simulink model "ExperimentalPowertrain"  (R2019b)
settings: Solver=ode1  StartTime=0.0  StopTime=inf  FixedStep=0.0002  RelTol=1e-3
PreLoadFcn:
  | vehicle = 'Car'; if ~length(which('cmself')), cmenv; end
  | ExperimentalPowertrain_bus
InitFcn:
  | vehicle = 'Car'; if ~length(which('cmself')), cmenv; end
  | ExperimentalPowertrain_bus
libraries: CarMaker4SL x8
(part 1 of 2)
Description:
  | CarMaker Plug-in Model Target
settings Model: Creator=caleb  LastModifiedBy=caleb
settings RTWCC: Description=CarMaker Plug-in Model Target  SystemTargetFile=CarMaker.tlc  TemplateMakefile=CarMaker_unix-win64.tmf
settings CodeAppCC: MaxIdLength=127
settings STFCustomTargetCC: TargetLangStandard=C99 (ISO)  CombineOutputUpdateFcns=on  MultiInstanceERTCode=on  CodeInterfacePackaging=Reusable function  GenerateAllocFcn=on  SystemTargetFile=CarMaker.tlc
settings GRTTargetCC: ParMdlRefBuildCompliant=off  CompOptLevelCompliant=off  ConcurrentExecutionCompliant=off  MatFileLogging=off  MultiInstanceERTCode=on  CodeInterfacePackaging=Reusable function  CPPClassGenCompliant=off  GenerateAllocFcn=on  UseToolchainInfoCompliant=off

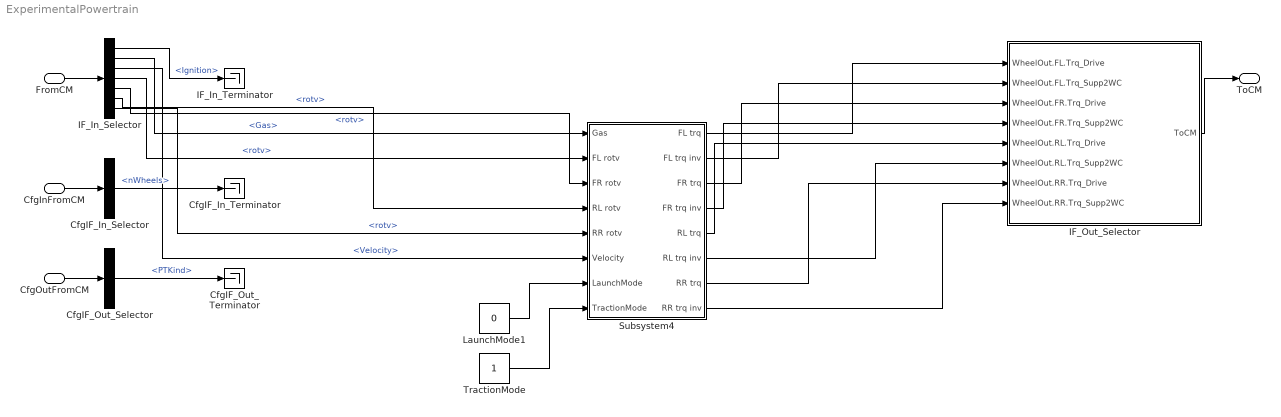
== system ExperimentalPowertrain ==
  FromCM : Inport  OutDataTypeStr=Bus: cmPowerTrainXWDIn
  CfgInFromCM : Inport  Port=2  OutDataTypeStr=Bus: cmPowerTrainXWDCfgIn
  CfgOutFromCM : Inport  Port=3  OutDataTypeStr=Bus: cmPowerTrainXWDCfgOut
  CfgIF_In_Selector : BusSelector  OutputSignals=nWheels
  CfgIF_In_Terminator : Terminator
  CfgIF_Out_Selector : BusSelector  OutputSignals=PTKind
  CfgIF_Out_Terminator : Terminator
  IF_In_Selector : BusSelector  OutputSignals=Ignition,Gas,Velocity,WheelIn.FL.rotv,WheelIn.FR.rotv,WheelIn.RL.rotv,WheelIn.RR.rotv
  IF_In_Terminator : Terminator
  IF_Out_Selector : Subsystem  mask(Signal Selection){}
      mask help: Signal Selection Block
      settings: OpenFcn=cmSignalSelect('SignalSelection_CB',gcb)
  LaunchMode1 : Constant  Value=0
  Subsystem4 : Subsystem
  TractionMode : Constant
  ToCM : Outport  OutDataTypeStr=Bus: cmPowerTrainXWDOut
  wires:
  FromCM/1 -> IF_In_Selector/1
  IF_In_Selector/1 -> IF_In_Terminator/1  "<Ignition>"
  IF_Out_Selector/1(ToCM) -> ToCM/1
  CfgInFromCM/1 -> CfgIF_In_Selector/1
  CfgIF_In_Selector/1 -> CfgIF_In_Terminator/1  "<nWheels>"
  CfgOutFromCM/1 -> CfgIF_Out_Selector/1
  CfgIF_Out_Selector/1 -> CfgIF_Out_Terminator/1  "<PTKind>"
  LaunchMode1/1 -> Subsystem4/7(LaunchMode)
  TractionMode/1 -> Subsystem4/8(TractionMode)
  IF_In_Selector/2 -> Subsystem4/1(Gas)  "<Gas>"
  IF_In_Selector/3 -> Subsystem4/6(Velocity)  "<Velocity>"
  IF_In_Selector/4 -> Subsystem4/2(FL rotv)  "<rotv>"
  IF_In_Selector/5 -> Subsystem4/3(FR rotv)  "<rotv>"
  IF_In_Selector/6 -> Subsystem4/4(RL rotv)  "<rotv>"
  IF_In_Selector/7 -> Subsystem4/5(RR rotv)  "<rotv>"
  Subsystem4/1(FL trq) -> IF_Out_Selector/1(WheelOut.FL.Trq_Drive)
  Subsystem4/2(FL trq inv) -> IF_Out_Selector/2(WheelOut.FL.Trq_Supp2WC)
  Subsystem4/3(FR trq) -> IF_Out_Selector/3(WheelOut.FR.Trq_Drive)
  Subsystem4/4(FR trq inv) -> IF_Out_Selector/4(WheelOut.FR.Trq_Supp2WC)
  Subsystem4/5(RL trq) -> IF_Out_Selector/5(WheelOut.RL.Trq_Drive)
  Subsystem4/6(RL trq inv) -> IF_Out_Selector/6(WheelOut.RL.Trq_Supp2WC)
  Subsystem4/7(RR trq) -> IF_Out_Selector/7(WheelOut.RR.Trq_Drive)
  Subsystem4/8(RR trq inv) -> IF_Out_Selector/8(WheelOut.RR.Trq_Supp2WC)

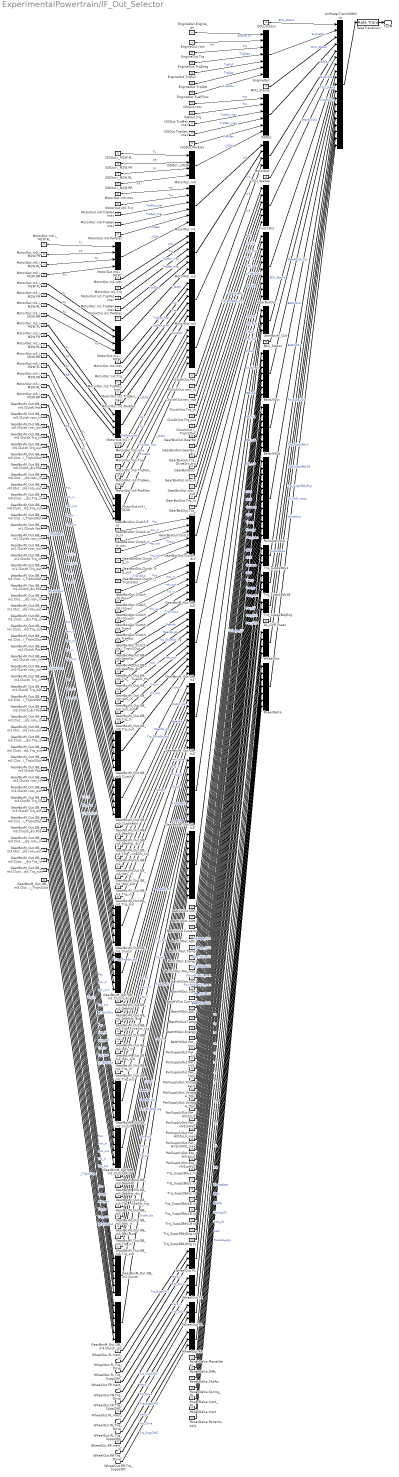
== system ExperimentalPowertrain/IF_Out_Selector ==
  WheelOut.FL.Trq_Drive : Inport
  WheelOut.FL.Trq_Supp2WC : Inport  Port=2
  WheelOut.FR.Trq_Drive : Inport  Port=3
  WheelOut.FR.Trq_Supp2WC : Inport  Port=4
  WheelOut.RL.Trq_Drive : Inport  Port=5
  WheelOut.RL.Trq_Supp2WC : Inport  Port=6
  WheelOut.RR.Trq_Drive : Inport  Port=7
  WheelOut.RR.Trq_Supp2WC : Inport  Port=8
  BCU_Status : Constant  Value=0
  BattHVOut : BusCreator  Inputs=7
  BattHVOut.AOC : Constant  Value=0
  BattHVOut.Current : Constant  Value=0
  BattHVOut.Energy : Constant  Value=0
  BattHVOut.Pwr_max : Constant  Value=0
  BattHVOut.SOC : Constant  Value=0
  BattHVOut.SOH : Constant  Value=0
  BattHVOut.Temp : Constant  Value=0
  BattLVOut : BusCreator  Inputs=7
  BattLVOut.AOC : Constant  Value=0
  BattLVOut.Current : Constant  Value=0
  BattLVOut.Energy : Constant  Value=0
  BattLVOut.Pwr_max : Constant  Value=0
  BattLVOut.SOC : Constant  Value=0
  BattLVOut.SOH : Constant  Value=0
  BattLVOut.Temp : Constant  Value=0
  ClutchOut : BusCreator  Inputs=6
  ClutchOut.Pos : Constant  Value=0
  ClutchOut.Trq_in : Constant  Value=0
  ClutchOut.Trq_out : Constant  Value=0
  ClutchOut.i_TrqIn2Out : Constant  Value=0
  ClutchOut.rotv_in : Constant  Value=0
  ClutchOut.rotv_out : Constant  Value=0
  DL_iDiff_mean : Constant  Value=0
  ECU_Status : Constant  Value=0
  EngineOut : BusCreator  Inputs=7
  EngineOut.Engine_on : Constant  Value=0
  EngineOut.FuelFlow : Constant  Value=0
  EngineOut.Trq : Constant  Value=0
  EngineOut.TrqDrag : Constant  Value=0
  EngineOut.TrqFull : Constant  Value=0
  EngineOut.TrqOpt : Constant  Value=0
  EngineOut.rotv : Constant  Value=0
  GearBoxM_Out : BusCreator  Inputs=4
  GearBoxM_Out.GB_m{0..3} (4 alike) : BusCreator  Inputs=10
  GearBoxM_Out.GB_m0.Clutch : BusCreator  Inputs=6
  GearBoxM_Out.GB_m0.Clutch.Pos : Constant  Value=0
  GearBoxM_Out.GB_m0.Clutch.Trq_in : Constant  Value=0
  GearBoxM_Out.GB_m0.Clutch.Trq_out : Constant  Value=0
  GearBoxM_Out.GB_m0.Clutch.i_TrqIn2Out : Constant  Value=0
  GearBoxM_Out.GB_m0.Clutch.rotv_in : Constant  Value=0
  GearBoxM_Out.GB_m0.Clutch.rotv_out : Constant  Value=0
  GearBoxM_Out.GB_m0.Clutch_dis : BusCreator  Inputs=6
  GearBoxM_Out.GB_m0.Clutch_dis.Pos : Constant  Value=0
  GearBoxM_Out.GB_m0.Clutch_dis.Trq_in : Constant  Value=0
  GearBoxM_Out.GB_m0.Clutch_dis.Trq_out : Constant  Value=0
  GearBoxM_Out.GB_m0.Clutch_dis.i_TrqIn2Out : Constant  Value=0
  GearBoxM_Out.GB_m0.Clutch_dis.rotv_in : Constant  Value=0
  GearBoxM_Out.GB_m0.Clutch_dis.rotv_out : Constant  Value=0
  GearBoxM_Out.GB_m0.GearNo : Constant  Value=0
  GearBoxM_Out.GB_m0.GearNo_dis : Constant  Value=0
  GearBoxM_Out.GB_m0.Trq_DriveSrc_trg : Constant  Value=0
  GearBoxM_Out.GB_m0.Trq_in : Constant  Value=0
  GearBoxM_Out.GB_m0.Trq_out : Constant  Value=0
  GearBoxM_Out.GB_m0.i : Constant  Value=0
  GearBoxM_Out.GB_m0.rotv_in : Constant  Value=0
  GearBoxM_Out.GB_m0.rotv_out : Constant  Value=0
  GearBoxM_Out.GB_m1.Clutch : BusCreator  Inputs=6
  GearBoxM_Out.GB_m1.Clutch.Pos : Constant  Value=0
  GearBoxM_Out.GB_m1.Clutch.Trq_in : Constant  Value=0
  GearBoxM_Out.GB_m1.Clutch.Trq_out : Constant  Value=0
  GearBoxM_Out.GB_m1.Clutch.i_TrqIn2Out : Constant  Value=0
  GearBoxM_Out.GB_m1.Clutch.rotv_in : Constant  Value=0
  GearBoxM_Out.GB_m1.Clutch.rotv_out : Constant  Value=0
  GearBoxM_Out.GB_m1.Clutch_dis : BusCreator  Inputs=6
  GearBoxM_Out.GB_m1.Clutch_dis.Pos : Constant  Value=0
  GearBoxM_Out.GB_m1.Clutch_dis.Trq_in : Constant  Value=0
  GearBoxM_Out.GB_m1.Clutch_dis.Trq_out : Constant  Value=0
  GearBoxM_Out.GB_m1.Clutch_dis.i_TrqIn2Out : Constant  Value=0
  GearBoxM_Out.GB_m1.Clutch_dis.rotv_in : Constant  Value=0
  GearBoxM_Out.GB_m1.Clutch_dis.rotv_out : Constant  Value=0
  GearBoxM_Out.GB_m1.GearNo : Constant  Value=0
  GearBoxM_Out.GB_m1.GearNo_dis : Constant  Value=0
  GearBoxM_Out.GB_m1.Trq_DriveSrc_trg : Constant  Value=0
  GearBoxM_Out.GB_m1.Trq_in : Constant  Value=0
  GearBoxM_Out.GB_m1.Trq_out : Constant  Value=0
  GearBoxM_Out.GB_m1.i : Constant  Value=0
  GearBoxM_Out.GB_m1.rotv_in : Constant  Value=0
  GearBoxM_Out.GB_m1.rotv_out : Constant  Value=0
  GearBoxM_Out.GB_m2.Clutch : BusCreator  Inputs=6
  GearBoxM_Out.GB_m2.Clutch.Pos : Constant  Value=0
  GearBoxM_Out.GB_m2.Clutch.Trq_in : Constant  Value=0
  GearBoxM_Out.GB_m2.Clutch.Trq_out : Constant  Value=0
  GearBoxM_Out.GB_m2.Clutch.i_TrqIn2Out : Constant  Value=0
  GearBoxM_Out.GB_m2.Clutch.rotv_in : Constant  Value=0
  GearBoxM_Out.GB_m2.Clutch.rotv_out : Constant  Value=0
  GearBoxM_Out.GB_m2.Clutch_dis : BusCreator  Inputs=6
  GearBoxM_Out.GB_m2.Clutch_dis.Pos : Constant  Value=0
  GearBoxM_Out.GB_m2.Clutch_dis.Trq_in : Constant  Value=0
  GearBoxM_Out.GB_m2.Clutch_dis.Trq_out : Constant  Value=0
  GearBoxM_Out.GB_m2.Clutch_dis.i_TrqIn2Out : Constant  Value=0
  GearBoxM_Out.GB_m2.Clutch_dis.rotv_in : Constant  Value=0
  GearBoxM_Out.GB_m2.Clutch_dis.rotv_out : Constant  Value=0
  GearBoxM_Out.GB_m2.GearNo : Constant  Value=0
  GearBoxM_Out.GB_m2.GearNo_dis : Constant  Value=0
  GearBoxM_Out.GB_m2.Trq_DriveSrc_trg : Constant  Value=0
  GearBoxM_Out.GB_m2.Trq_in : Constant  Value=0
  GearBoxM_Out.GB_m2.Trq_out : Constant  Value=0
  GearBoxM_Out.GB_m2.i : Constant  Value=0
  GearBoxM_Out.GB_m2.rotv_in : Constant  Value=0
  GearBoxM_Out.GB_m2.rotv_out : Constant  Value=0
  GearBoxM_Out.GB_m3.Clutch : BusCreator  Inputs=6
  GearBoxM_Out.GB_m3.Clutch.Pos : Constant  Value=0
  GearBoxM_Out.GB_m3.Clutch.Trq_in : Constant  Value=0
  GearBoxM_Out.GB_m3.Clutch.Trq_out : Constant  Value=0
  GearBoxM_Out.GB_m3.Clutch.i_TrqIn2Out : Constant  Value=0
  GearBoxM_Out.GB_m3.Clutch.rotv_in : Constant  Value=0
  GearBoxM_Out.GB_m3.Clutch.rotv_out : Constant  Value=0
  GearBoxM_Out.GB_m3.Clutch_dis : BusCreator  Inputs=6
  GearBoxM_Out.GB_m3.Clutch_dis.Pos : Constant  Value=0
  GearBoxM_Out.GB_m3.Clutch_dis.Trq_in : Constant  Value=0
  GearBoxM_Out.GB_m3.Clutch_dis.Trq_out : Constant  Value=0
  GearBoxM_Out.GB_m3.Clutch_dis.i_TrqIn2Out : Constant  Value=0
  GearBoxM_Out.GB_m3.Clutch_dis.rotv_in : Constant  Value=0
  GearBoxM_Out.GB_m3.Clutch_dis.rotv_out : Constant  Value=0
  GearBoxM_Out.GB_m3.GearNo : Constant  Value=0
  GearBoxM_Out.GB_m3.GearNo_dis : Constant  Value=0
  GearBoxM_Out.GB_m3.Trq_DriveSrc_trg : Constant  Value=0
  GearBoxM_Out.GB_m3.Trq_in : Constant  Value=0
  GearBoxM_Out.GB_m3.Trq_out : Constant  Value=0
  GearBoxM_Out.GB_m3.i : Constant  Value=0
  GearBoxM_Out.GB_m3.rotv_in : Constant  Value=0
  GearBoxM_Out.GB_m3.rotv_out : Constant  Value=0
  GearBoxOut : BusCreator  Inputs=10
  GearBoxOut.Clutch : BusCreator  Inputs=6
  GearBoxOut.Clutch.Pos : Constant  Value=0
  GearBoxOut.Clutch.Trq_in : Constant  Value=0
  GearBoxOut.Clutch.Trq_out : Constant  Value=0
  GearBoxOut.Clutch.i_TrqIn2Out : Constant  Value=0
  GearBoxOut.Clutch.rotv_in : Constant  Value=0
  GearBoxOut.Clutch.rotv_out : Constant  Value=0
  GearBoxOut.Clutch_dis : BusCreator  Inputs=6
  GearBoxOut.Clutch_dis.Pos : Constant  Value=0
  GearBoxOut.Clutch_dis.Trq_in : Constant  Value=0
  GearBoxOut.Clutch_dis.Trq_out : Constant  Value=0
  GearBoxOut.Clutch_dis.i_TrqIn2Out : Constant  Value=0
  GearBoxOut.Clutch_dis.rotv_in : Constant  Value=0
  GearBoxOut.Clutch_dis.rotv_out : Constant  Value=0
  GearBoxOut.GearNo : Constant  Value=0
  GearBoxOut.GearNo_dis : Constant  Value=0
  GearBoxOut.Trq_DriveSrc_trg : Constant  Value=0
  GearBoxOut.Trq_in : Constant  Value=0
  GearBoxOut.Trq_out : Constant  Value=0
  GearBoxOut.i : Constant  Value=0
  GearBoxOut.rotv_in : Constant  Value=0
  GearBoxOut.rotv_out : Constant  Value=0
  ISGOut : BusCreator  Inputs=6
  ISGOut.PwrElec : Constant  Value=0
  ISGOut.Trq : Constant  Value=0
  ISGOut.TrqGen_max : Constant  Value=0
  ISGOut.TrqMot_max : Constant  Value=0
  ISGOut.i_M2W : BusCreator  Inputs=4
  ISGOut.i_M2W.FL : Constant  Value=0
  ISGOut.i_M2W.FR : Constant  Value=0
  ISGOut.i_M2W.RL : Constant  Value=0
  ISGOut.i_M2W.RR : Constant  Value=0
  ISGOut.rotv : Constant  Value=0
  MCU_Status : Constant  Value=0
  MotorOut : BusCreator  Inputs=4
  MotorOut.m{0..3} (4 alike) : BusCreator  Inputs=6
  MotorOut.m0.PwrElec : Constant  Value=0
  MotorOut.m0.Trq : Constant  Value=0
  MotorOut.m0.TrqGen_max : Constant  Value=0
  MotorOut.m0.TrqMot_max : Constant  Value=0
  MotorOut.m0.i_M2W : BusCreator  Inputs=4
  MotorOut.m0.i_M2W.FL : Constant  Value=0
  MotorOut.m0.i_M2W.FR : Constant  Value=0
  MotorOut.m0.i_M2W.RL : Constant  Value=0
  MotorOut.m0.i_M2W.RR : Constant  Value=0
  MotorOut.m0.rotv : Constant  Value=0
  MotorOut.m1.PwrElec : Constant  Value=0
  MotorOut.m1.Trq : Constant  Value=0
  MotorOut.m1.TrqGen_max : Constant  Value=0
  MotorOut.m1.TrqMot_max : Constant  Value=0
  MotorOut.m1.i_M2W : BusCreator  Inputs=4
  MotorOut.m1.i_M2W.FL : Constant  Value=0
  MotorOut.m1.i_M2W.FR : Constant  Value=0
  MotorOut.m1.i_M2W.RL : Constant  Value=0
  MotorOut.m1.i_M2W.RR : Constant  Value=0
  MotorOut.m1.rotv : Constant  Value=0
  MotorOut.m2.PwrElec : Constant  Value=0
  MotorOut.m2.Trq : Constant  Value=0
  MotorOut.m2.TrqGen_max : Constant  Value=0
  MotorOut.m2.TrqMot_max : Constant  Value=0
  MotorOut.m2.i_M2W : BusCreator  Inputs=4
  MotorOut.m2.i_M2W.FL : Constant  Value=0
  MotorOut.m2.i_M2W.FR : Constant  Value=0
  MotorOut.m2.i_M2W.RL : Constant  Value=0
  MotorOut.m2.i_M2W.RR : Constant  Value=0
  MotorOut.m2.rotv : Constant  Value=0
  MotorOut.m3.PwrElec : Constant  Value=0
  MotorOut.m3.Trq : Constant  Value=0
  MotorOut.m3.TrqGen_max : Constant  Value=0
  MotorOut.m3.TrqMot_max : Constant  Value=0
  MotorOut.m3.i_M2W : BusCreator  Inputs=4
  MotorOut.m3.i_M2W.FL : Constant  Value=0
  MotorOut.m3.i_M2W.FR : Constant  Value=0
  MotorOut.m3.i_M2W.RL : Constant  Value=0
  MotorOut.m3.i_M2W.RR : Constant  Value=0
  MotorOut.m3.rotv : Constant  Value=0
  PowerDelta : BusCreator  Inputs=7
  PowerDelta.Diffs : Constant  Value=0
  PowerDelta.Inert : Constant  Value=0
  PowerDelta.Inert_DL : Constant  Value=0
  PowerDelta.PlanetGear : Constant  Value=0
  PowerDelta.PowerSupply : Constant  Value=0
  PowerDelta.Shafts : Constant  Value=0
  PowerDelta.Spring_DL : Constant  Value=0
  PwrSupplyOut : BusCreator  Inputs=12
  PwrSupplyOut.Eta_HV1toHV2 : Constant  Value=0
  PwrSupplyOut.Eta_HV1toLV : Constant  Value=0
  PwrSupplyOut.Pwr_HV1 : Constant  Value=0
  PwrSupplyOut.Pwr_HV1toHV2 : Constant  Value=0
  PwrSupplyOut.Pwr_HV1toHV2_max : Constant  Value=0
  PwrSupplyOut.Pwr_HV1toLV : Constant  Value=0
  PwrSupplyOut.Pwr_HV1toLV_max : Constant  Value=0
  PwrSupplyOut.Pwr_HV2 : Constant  Value=0
  PwrSupplyOut.Pwr_LV : Constant  Value=0
  PwrSupplyOut.Voltage_HV1 : Constant  Value=0
  PwrSupplyOut.Voltage_HV2 : Constant  Value=0
  PwrSupplyOut.Voltage_LV : Constant  Value=0
  RateTransition : RateTransition  OutPortSampleTime=str2num(get_param(bdroot,'FixedStep'))
  TCU_Status : Constant  Value=0
  Trq_Supp2Bdy1 : BusCreator  Inputs=3
  Trq_Supp2Bdy1.rx : Constant  Value=0
  Trq_Supp2Bdy1.ry : Constant  Value=0
  Trq_Supp2Bdy1.rz : Constant  Value=0
  Trq_Supp2Bdy1B : BusCreator  Inputs=3
  Trq_Supp2Bdy1B.rx : Constant  Value=0
  Trq_Supp2Bdy1B.ry : Constant  Value=0
  Trq_Supp2Bdy1B.rz : Constant  Value=0
  Trq_Supp2BdyEng : BusCreator  Inputs=2
  Trq_Supp2BdyEng.rx : Constant  Value=0
  Trq_Supp2BdyEng.ry : Constant  Value=0
  WheelOut : BusCreator  Inputs=4
  WheelOut.FL : BusCreator  Inputs=3
  WheelOut.FL.Inert_in : Constant  Value=0
  WheelOut.FR : BusCreator  Inputs=3
  WheelOut.FR.Inert_in : Constant  Value=0
  WheelOut.RL : BusCreator  Inputs=3
  WheelOut.RL.Inert_in : Constant  Value=0
  WheelOut.RR : BusCreator  Inputs=3
  WheelOut.RR.Inert_in : Constant  Value=0
  cmPowerTrainXWDOut : BusCreator  Inputs=19
  ToCM : Outport
  wires:
  RateTransition/1 -> ToCM/1
  cmPowerTrainXWDOut/1 -> RateTransition/1
  ECU_Status/1 -> cmPowerTrainXWDOut/1  "ECU_Status"
  EngineOut/1 -> cmPowerTrainXWDOut/2  "EngineOut"
  EngineOut.Engine_on/1 -> EngineOut/1  "Engine_on"
  EngineOut.rotv/1 -> EngineOut/2  "rotv"
  EngineOut.Trq/1 -> EngineOut/3  "Trq"
  EngineOut.TrqDrag/1 -> EngineOut/4  "TrqDrag"
  EngineOut.TrqFull/1 -> EngineOut/5  "TrqFull"
  EngineOut.TrqOpt/1 -> EngineOut/6  "TrqOpt"
  EngineOut.FuelFlow/1 -> EngineOut/7  "FuelFlow"
  MCU_Status/1 -> cmPowerTrainXWDOut/3  "MCU_Status"
  ISGOut/1 -> cmPowerTrainXWDOut/4  "ISGOut"
  ISGOut.rotv/1 -> ISGOut/1  "rotv"
  ISGOut.Trq/1 -> ISGOut/2  "Trq"
  ISGOut.TrqMot_max/1 -> ISGOut/3  "TrqMot_max"
  ISGOut.TrqGen_max/1 -> ISGOut/4  "TrqGen_max"
  ISGOut.PwrElec/1 -> ISGOut/5  "PwrElec"
  ISGOut.i_M2W/1 -> ISGOut/6  "i_M2W"
  ISGOut.i_M2W.FL/1 -> ISGOut.i_M2W/1  "FL"
  ISGOut.i_M2W.FR/1 -> ISGOut.i_M2W/2  "FR"
  ISGOut.i_M2W.RL/1 -> ISGOut.i_M2W/3  "RL"
  ISGOut.i_M2W.RR/1 -> ISGOut.i_M2W/4  "RR"
  MotorOut/1 -> cmPowerTrainXWDOut/5  "MotorOut"
  MotorOut.m0/1 -> MotorOut/1  "m0"
  MotorOut.m0.rotv/1 -> MotorOut.m0/1  "rotv"
  MotorOut.m0.Trq/1 -> MotorOut.m0/2  "Trq"
  MotorOut.m0.TrqMot_max/1 -> MotorOut.m0/3  "TrqMot_max"
  MotorOut.m0.TrqGen_max/1 -> MotorOut.m0/4  "TrqGen_max"
  MotorOut.m0.PwrElec/1 -> MotorOut.m0/5  "PwrElec"
  MotorOut.m0.i_M2W/1 -> MotorOut.m0/6  "i_M2W"
  MotorOut.m0.i_M2W.FL/1 -> MotorOut.m0.i_M2W/1  "FL"
  MotorOut.m0.i_M2W.FR/1 -> MotorOut.m0.i_M2W/2  "FR"
  MotorOut.m0.i_M2W.RL/1 -> MotorOut.m0.i_M2W/3  "RL"
  MotorOut.m0.i_M2W.RR/1 -> MotorOut.m0.i_M2W/4  "RR"
  MotorOut.m1/1 -> MotorOut/2  "m1"
  MotorOut.m1.rotv/1 -> MotorOut.m1/1  "rotv"
  MotorOut.m1.Trq/1 -> MotorOut.m1/2  "Trq"
  MotorOut.m1.TrqMot_max/1 -> MotorOut.m1/3  "TrqMot_max"
  MotorOut.m1.TrqGen_max/1 -> MotorOut.m1/4  "TrqGen_max"
  MotorOut.m1.PwrElec/1 -> MotorOut.m1/5  "PwrElec"
  MotorOut.m1.i_M2W/1 -> MotorOut.m1/6  "i_M2W"
  MotorOut.m1.i_M2W.FL/1 -> MotorOut.m1.i_M2W/1  "FL"
  MotorOut.m1.i_M2W.FR/1 -> MotorOut.m1.i_M2W/2  "FR"
  MotorOut.m1.i_M2W.RL/1 -> MotorOut.m1.i_M2W/3  "RL"
  MotorOut.m1.i_M2W.RR/1 -> MotorOut.m1.i_M2W/4  "RR"
  MotorOut.m2/1 -> MotorOut/3  "m2"
  MotorOut.m2.rotv/1 -> MotorOut.m2/1  "rotv"
  MotorOut.m2.Trq/1 -> MotorOut.m2/2  "Trq"
  MotorOut.m2.TrqMot_max/1 -> MotorOut.m2/3  "TrqMot_max"
  MotorOut.m2.TrqGen_max/1 -> MotorOut.m2/4  "TrqGen_max"
  MotorOut.m2.PwrElec/1 -> MotorOut.m2/5  "PwrElec"
  MotorOut.m2.i_M2W/1 -> MotorOut.m2/6  "i_M2W"
  MotorOut.m2.i_M2W.FL/1 -> MotorOut.m2.i_M2W/1  "FL"
  MotorOut.m2.i_M2W.FR/1 -> MotorOut.m2.i_M2W/2  "FR"
  MotorOut.m2.i_M2W.RL/1 -> MotorOut.m2.i_M2W/3  "RL"
  MotorOut.m2.i_M2W.RR/1 -> MotorOut.m2.i_M2W/4  "RR"
  MotorOut.m3/1 -> MotorOut/4  "m3"
  MotorOut.m3.rotv/1 -> MotorOut.m3/1  "rotv"
  MotorOut.m3.Trq/1 -> MotorOut.m3/2  "Trq"
  MotorOut.m3.TrqMot_max/1 -> MotorOut.m3/3  "TrqMot_max"
  MotorOut.m3.TrqGen_max/1 -> MotorOut.m3/4  "TrqGen_max"
  MotorOut.m3.PwrElec/1 -> MotorOut.m3/5  "PwrElec"
  MotorOut.m3.i_M2W/1 -> MotorOut.m3/6  "i_M2W"
  MotorOut.m3.i_M2W.FL/1 -> MotorOut.m3.i_M2W/1  "FL"
  MotorOut.m3.i_M2W.FR/1 -> MotorOut.m3.i_M2W/2  "FR"
  MotorOut.m3.i_M2W.RL/1 -> MotorOut.m3.i_M2W/3  "RL"
  MotorOut.m3.i_M2W.RR/1 -> MotorOut.m3.i_M2W/4  "RR"
  TCU_Status/1 -> cmPowerTrainXWDOut/6  "TCU_Status"
  ClutchOut/1 -> cmPowerTrainXWDOut/7  "ClutchOut"
  ClutchOut.Pos/1 -> ClutchOut/1  "Pos"
  ClutchOut.rotv_in/1 -> ClutchOut/2  "rotv_in"
  ClutchOut.rotv_out/1 -> ClutchOut/3  "rotv_out"
  ClutchOut.Trq_in/1 -> ClutchOut/4  "Trq_in"
  ClutchOut.Trq_out/1 -> ClutchOut/5  "Trq_out"
  ClutchOut.i_TrqIn2Out/1 -> ClutchOut/6  "i_TrqIn2Out"
  GearBoxOut/1 -> cmPowerTrainXWDOut/8  "GearBoxOut"
  GearBoxOut.GearNo/1 -> GearBoxOut/1  "GearNo"
  GearBoxOut.GearNo_dis/1 -> GearBoxOut/2  "GearNo_dis"
  GearBoxOut.Trq_DriveSrc_trg/1 -> GearBoxOut/3  "Trq_DriveSrc_trg"
  GearBoxOut.i/1 -> GearBoxOut/4  "i"
  GearBoxOut.rotv_in/1 -> GearBoxOut/5  "rotv_in"
  GearBoxOut.rotv_out/1 -> GearBoxOut/6  "rotv_out"
  GearBoxOut.Trq_in/1 -> GearBoxOut/7  "Trq_in"
  GearBoxOut.Trq_out/1 -> GearBoxOut/8  "Trq_out"
  GearBoxOut.Clutch/1 -> GearBoxOut/9  "Clutch"
  GearBoxOut.Clutch.Pos/1 -> GearBoxOut.Clutch/1  "Pos"
  GearBoxOut.Clutch.rotv_in/1 -> GearBoxOut.Clutch/2  "rotv_in"
  GearBoxOut.Clutch.rotv_out/1 -> GearBoxOut.Clutch/3  "rotv_out"
  GearBoxOut.Clutch.Trq_in/1 -> GearBoxOut.Clutch/4  "Trq_in"
  GearBoxOut.Clutch.Trq_out/1 -> GearBoxOut.Clutch/5  "Trq_out"
  GearBoxOut.Clutch.i_TrqIn2Out/1 -> GearBoxOut.Clutch/6  "i_TrqIn2Out"
  GearBoxOut.Clutch_dis/1 -> GearBoxOut/10  "Clutch_dis"
  GearBoxOut.Clutch_dis.Pos/1 -> GearBoxOut.Clutch_dis/1  "Pos"
  GearBoxOut.Clutch_dis.rotv_in/1 -> GearBoxOut.Clutch_dis/2  "rotv_in"
  GearBoxOut.Clutch_dis.rotv_out/1 -> GearBoxOut.Clutch_dis/3  "rotv_out"
  GearBoxOut.Clutch_dis.Trq_in/1 -> GearBoxOut.Clutch_dis/4  "Trq_in"
  GearBoxOut.Clutch_dis.Trq_out/1 -> GearBoxOut.Clutch_dis/5  "Trq_out"
  GearBoxOut.Clutch_dis.i_TrqIn2Out/1 -> GearBoxOut.Clutch_dis/6  "i_TrqIn2Out"
  GearBoxM_Out/1 -> cmPowerTrainXWDOut/9  "GearBoxM_Out"
  GearBoxM_Out.GB_m0/1 -> GearBoxM_Out/1  "GB_m0"
  GearBoxM_Out.GB_m0.GearNo/1 -> GearBoxM_Out.GB_m0/1  "GearNo"
  GearBoxM_Out.GB_m0.GearNo_dis/1 -> GearBoxM_Out.GB_m0/2  "GearNo_dis"
  GearBoxM_Out.GB_m0.Trq_DriveSrc_trg/1 -> GearBoxM_Out.GB_m0/3  "Trq_DriveSrc_trg"
  GearBoxM_Out.GB_m0.i/1 -> GearBoxM_Out.GB_m0/4  "i"
  GearBoxM_Out.GB_m0.rotv_in/1 -> GearBoxM_Out.GB_m0/5  "rotv_in"
  GearBoxM_Out.GB_m0.rotv_out/1 -> GearBoxM_Out.GB_m0/6  "rotv_out"
  GearBoxM_Out.GB_m0.Trq_in/1 -> GearBoxM_Out.GB_m0/7  "Trq_in"
  GearBoxM_Out.GB_m0.Trq_out/1 -> GearBoxM_Out.GB_m0/8  "Trq_out"
  GearBoxM_Out.GB_m0.Clutch/1 -> GearBoxM_Out.GB_m0/9  "Clutch"
  GearBoxM_Out.GB_m0.Clutch.Pos/1 -> GearBoxM_Out.GB_m0.Clutch/1  "Pos"
  GearBoxM_Out.GB_m0.Clutch.rotv_in/1 -> GearBoxM_Out.GB_m0.Clutch/2  "rotv_in"
  GearBoxM_Out.GB_m0.Clutch.rotv_out/1 -> GearBoxM_Out.GB_m0.Clutch/3  "rotv_out"
  GearBoxM_Out.GB_m0.Clutch.Trq_in/1 -> GearBoxM_Out.GB_m0.Clutch/4  "Trq_in"
  GearBoxM_Out.GB_m0.Clutch.Trq_out/1 -> GearBoxM_Out.GB_m0.Clutch/5  "Trq_out"
  GearBoxM_Out.GB_m0.Clutch.i_TrqIn2Out/1 -> GearBoxM_Out.GB_m0.Clutch/6  "i_TrqIn2Out"
  GearBoxM_Out.GB_m0.Clutch_dis/1 -> GearBoxM_Out.GB_m0/10  "Clutch_dis"
  GearBoxM_Out.GB_m0.Clutch_dis.Pos/1 -> GearBoxM_Out.GB_m0.Clutch_dis/1  "Pos"
  GearBoxM_Out.GB_m0.Clutch_dis.rotv_in/1 -> GearBoxM_Out.GB_m0.Clutch_dis/2  "rotv_in"
  GearBoxM_Out.GB_m0.Clutch_dis.rotv_out/1 -> GearBoxM_Out.GB_m0.Clutch_dis/3  "rotv_out"
  GearBoxM_Out.GB_m0.Clutch_dis.Trq_in/1 -> GearBoxM_Out.GB_m0.Clutch_dis/4  "Trq_in"
  GearBoxM_Out.GB_m0.Clutch_dis.Trq_out/1 -> GearBoxM_Out.GB_m0.Clutch_dis/5  "Trq_out"
  GearBoxM_Out.GB_m0.Clutch_dis.i_TrqIn2Out/1 -> GearBoxM_Out.GB_m0.Clutch_dis/6  "i_TrqIn2Out"
  GearBoxM_Out.GB_m1/1 -> GearBoxM_Out/2  "GB_m1"
  GearBoxM_Out.GB_m1.GearNo/1 -> GearBoxM_Out.GB_m1/1  "GearNo"
  GearBoxM_Out.GB_m1.GearNo_dis/1 -> GearBoxM_Out.GB_m1/2  "GearNo_dis"
  GearBoxM_Out.GB_m1.Trq_DriveSrc_trg/1 -> GearBoxM_Out.GB_m1/3  "Trq_DriveSrc_trg"
  GearBoxM_Out.GB_m1.i/1 -> GearBoxM_Out.GB_m1/4  "i"
  GearBoxM_Out.GB_m1.rotv_in/1 -> GearBoxM_Out.GB_m1/5  "rotv_in"
  GearBoxM_Out.GB_m1.rotv_out/1 -> GearBoxM_Out.GB_m1/6  "rotv_out"
  GearBoxM_Out.GB_m1.Trq_in/1 -> GearBoxM_Out.GB_m1/7  "Trq_in"
  GearBoxM_Out.GB_m1.Trq_out/1 -> GearBoxM_Out.GB_m1/8  "Trq_out"
  GearBoxM_Out.GB_m1.Clutch/1 -> GearBoxM_Out.GB_m1/9  "Clutch"
  GearBoxM_Out.GB_m1.Clutch.Pos/1 -> GearBoxM_Out.GB_m1.Clutch/1  "Pos"
  GearBoxM_Out.GB_m1.Clutch.rotv_in/1 -> GearBoxM_Out.GB_m1.Clutch/2  "rotv_in"
  GearBoxM_Out.GB_m1.Clutch.rotv_out/1 -> GearBoxM_Out.GB_m1.Clutch/3  "rotv_out"
  GearBoxM_Out.GB_m1.Clutch.Trq_in/1 -> GearBoxM_Out.GB_m1.Clutch/4  "Trq_in"
  GearBoxM_Out.GB_m1.Clutch.Trq_out/1 -> GearBoxM_Out.GB_m1.Clutch/5  "Trq_out"
  GearBoxM_Out.GB_m1.Clutch.i_TrqIn2Out/1 -> GearBoxM_Out.GB_m1.Clutch/6  "i_TrqIn2Out"
  GearBoxM_Out.GB_m1.Clutch_dis/1 -> GearBoxM_Out.GB_m1/10  "Clutch_dis"
  GearBoxM_Out.GB_m1.Clutch_dis.Pos/1 -> GearBoxM_Out.GB_m1.Clutch_dis/1  "Pos"
  GearBoxM_Out.GB_m1.Clutch_dis.rotv_in/1 -> GearBoxM_Out.GB_m1.Clutch_dis/2  "rotv_in"
  GearBoxM_Out.GB_m1.Clutch_dis.rotv_out/1 -> GearBoxM_Out.GB_m1.Clutch_dis/3  "rotv_out"
  GearBoxM_Out.GB_m1.Clutch_dis.Trq_in/1 -> GearBoxM_Out.GB_m1.Clutch_dis/4  "Trq_in"
  GearBoxM_Out.GB_m1.Clutch_dis.Trq_out/1 -> GearBoxM_Out.GB_m1.Clutch_dis/5  "Trq_out"
  GearBoxM_Out.GB_m1.Clutch_dis.i_TrqIn2Out/1 -> GearBoxM_Out.GB_m1.Clutch_dis/6  "i_TrqIn2Out"
  GearBoxM_Out.GB_m2/1 -> GearBoxM_Out/3  "GB_m2"
  GearBoxM_Out.GB_m2.GearNo/1 -> GearBoxM_Out.GB_m2/1  "GearNo"
  GearBoxM_Out.GB_m2.GearNo_dis/1 -> GearBoxM_Out.GB_m2/2  "GearNo_dis"
  GearBoxM_Out.GB_m2.Trq_DriveSrc_trg/1 -> GearBoxM_Out.GB_m2/3  "Trq_DriveSrc_trg"
  GearBoxM_Out.GB_m2.i/1 -> GearBoxM_Out.GB_m2/4  "i"
  GearBoxM_Out.GB_m2.rotv_in/1 -> GearBoxM_Out.GB_m2/5  "rotv_in"
  GearBoxM_Out.GB_m2.rotv_out/1 -> GearBoxM_Out.GB_m2/6  "rotv_out"
  GearBoxM_Out.GB_m2.Trq_in/1 -> GearBoxM_Out.GB_m2/7  "Trq_in"
  GearBoxM_Out.GB_m2.Trq_out/1 -> GearBoxM_Out.GB_m2/8  "Trq_out"
  GearBoxM_Out.GB_m2.Clutch/1 -> GearBoxM_Out.GB_m2/9  "Clutch"
  GearBoxM_Out.GB_m2.Clutch.Pos/1 -> GearBoxM_Out.GB_m2.Clutch/1  "Pos"
  GearBoxM_Out.GB_m2.Clutch.rotv_in/1 -> GearBoxM_Out.GB_m2.Clutch/2  "rotv_in"
  GearBoxM_Out.GB_m2.Clutch.rotv_out/1 -> GearBoxM_Out.GB_m2.Clutch/3  "rotv_out"
  GearBoxM_Out.GB_m2.Clutch.Trq_in/1 -> GearBoxM_Out.GB_m2.Clutch/4  "Trq_in"
  GearBoxM_Out.GB_m2.Clutch.Trq_out/1 -> GearBoxM_Out.GB_m2.Clutch/5  "Trq_out"
  GearBoxM_Out.GB_m2.Clutch.i_TrqIn2Out/1 -> GearBoxM_Out.GB_m2.Clutch/6  "i_TrqIn2Out"
  GearBoxM_Out.GB_m2.Clutch_dis/1 -> GearBoxM_Out.GB_m2/10  "Clutch_dis"
  GearBoxM_Out.GB_m2.Clutch_dis.Pos/1 -> GearBoxM_Out.GB_m2.Clutch_dis/1  "Pos"
  GearBoxM_Out.GB_m2.Clutch_dis.rotv_in/1 -> GearBoxM_Out.GB_m2.Clutch_dis/2  "rotv_in"
  GearBoxM_Out.GB_m2.Clutch_dis.rotv_out/1 -> GearBoxM_Out.GB_m2.Clutch_dis/3  "rotv_out"
  GearBoxM_Out.GB_m2.Clutch_dis.Trq_in/1 -> GearBoxM_Out.GB_m2.Clutch_dis/4  "Trq_in"
  GearBoxM_Out.GB_m2.Clutch_dis.Trq_out/1 -> GearBoxM_Out.GB_m2.Clutch_dis/5  "Trq_out"
  GearBoxM_Out.GB_m2.Clutch_dis.i_TrqIn2Out/1 -> GearBoxM_Out.GB_m2.Clutch_dis/6  "i_TrqIn2Out"
  GearBoxM_Out.GB_m3/1 -> GearBoxM_Out/4  "GB_m3"
  GearBoxM_Out.GB_m3.GearNo/1 -> GearBoxM_Out.GB_m3/1  "GearNo"
  GearBoxM_Out.GB_m3.GearNo_dis/1 -> GearBoxM_Out.GB_m3/2  "GearNo_dis"
  GearBoxM_Out.GB_m3.Trq_DriveSrc_trg/1 -> GearBoxM_Out.GB_m3/3  "Trq_DriveSrc_trg"
  GearBoxM_Out.GB_m3.i/1 -> GearBoxM_Out.GB_m3/4  "i"
  GearBoxM_Out.GB_m3.rotv_in/1 -> GearBoxM_Out.GB_m3/5  "rotv_in"
  GearBoxM_Out.GB_m3.rotv_out/1 -> GearBoxM_Out.GB_m3/6  "rotv_out"
  GearBoxM_Out.GB_m3.Trq_in/1 -> GearBoxM_Out.GB_m3/7  "Trq_in"
  GearBoxM_Out.GB_m3.Trq_out/1 -> GearBoxM_Out.GB_m3/8  "Trq_out"
  GearBoxM_Out.GB_m3.Clutch/1 -> GearBoxM_Out.GB_m3/9  "Clutch"
  GearBoxM_Out.GB_m3.Clutch.Pos/1 -> GearBoxM_Out.GB_m3.Clutch/1  "Pos"
  GearBoxM_Out.GB_m3.Clutch.rotv_in/1 -> GearBoxM_Out.GB_m3.Clutch/2  "rotv_in"
  GearBoxM_Out.GB_m3.Clutch.rotv_out/1 -> GearBoxM_Out.GB_m3.Clutch/3  "rotv_out"
  GearBoxM_Out.GB_m3.Clutch.Trq_in/1 -> GearBoxM_Out.GB_m3.Clutch/4  "Trq_in"
  GearBoxM_Out.GB_m3.Clutch.Trq_out/1 -> GearBoxM_Out.GB_m3.Clutch/5  "Trq_out"
  GearBoxM_Out.GB_m3.Clutch.i_TrqIn2Out/1 -> GearBoxM_Out.GB_m3.Clutch/6  "i_TrqIn2Out"
  GearBoxM_Out.GB_m3.Clutch_dis/1 -> GearBoxM_Out.GB_m3/10  "Clutch_dis"
  GearBoxM_Out.GB_m3.Clutch_dis.Pos/1 -> GearBoxM_Out.GB_m3.Clutch_dis/1  "Pos"
  GearBoxM_Out.GB_m3.Clutch_dis.rotv_in/1 -> GearBoxM_Out.GB_m3.Clutch_dis/2  "rotv_in"
  GearBoxM_Out.GB_m3.Clutch_dis.rotv_out/1 -> GearBoxM_Out.GB_m3.Clutch_dis/3  "rotv_out"
  GearBoxM_Out.GB_m3.Clutch_dis.Trq_in/1 -> GearBoxM_Out.GB_m3.Clutch_dis/4  "Trq_in"
  GearBoxM_Out.GB_m3.Clutch_dis.Trq_out/1 -> GearBoxM_Out.GB_m3.Clutch_dis/5  "Trq_out"
  GearBoxM_Out.GB_m3.Clutch_dis.i_TrqIn2Out/1 -> GearBoxM_Out.GB_m3.Clutch_dis/6  "i_TrqIn2Out"
  BCU_Status/1 -> cmPowerTrainXWDOut/10  "BCU_Status"
  BattLVOut/1 -> cmPowerTrainXWDOut/11  "BattLVOut"
  BattLVOut.SOC/1 -> BattLVOut/1  "SOC"
  BattLVOut.SOH/1 -> BattLVOut/2  "SOH"
  BattLVOut.Current/1 -> BattLVOut/3  "Current"
  BattLVOut.AOC/1 -> BattLVOut/4  "AOC"
  BattLVOut.Temp/1 -> BattLVOut/5  "Temp"
  BattLVOut.Energy/1 -> BattLVOut/6  "Energy"
  BattLVOut.Pwr_max/1 -> BattLVOut/7  "Pwr_max"
  BattHVOut/1 -> cmPowerTrainXWDOut/12  "BattHVOut"
  BattHVOut.SOC/1 -> BattHVOut/1  "SOC"
  BattHVOut.SOH/1 -> BattHVOut/2  "SOH"
  BattHVOut.Current/1 -> BattHVOut/3  "Current"
  BattHVOut.AOC/1 -> BattHVOut/4  "AOC"
  BattHVOut.Temp/1 -> BattHVOut/5  "Temp"
  BattHVOut.Energy/1 -> BattHVOut/6  "Energy"
  BattHVOut.Pwr_max/1 -> BattHVOut/7  "Pwr_max"
  PwrSupplyOut/1 -> cmPowerTrainXWDOut/13  "PwrSupplyOut"
  PwrSupplyOut.Pwr_LV/1 -> PwrSupplyOut/1  "Pwr_LV"
  PwrSupplyOut.Pwr_HV1/1 -> PwrSupplyOut/2  "Pwr_HV1"
  PwrSupplyOut.Pwr_HV2/1 -> PwrSupplyOut/3  "Pwr_HV2"
  PwrSupplyOut.Voltage_LV/1 -> PwrSupplyOut/4  "Voltage_LV"
  PwrSupplyOut.Voltage_HV1/1 -> PwrSupplyOut/5  "Voltage_HV1"
  PwrSupplyOut.Voltage_HV2/1 -> PwrSupplyOut/6  "Voltage_HV2"
  PwrSupplyOut.Pwr_HV1toLV/1 -> PwrSupplyOut/7  "Pwr_HV1toLV"
  PwrSupplyOut.Pwr_HV1toHV2/1 -> PwrSupplyOut/8  "Pwr_HV1toHV2"
  PwrSupplyOut.Pwr_HV1toLV_max/1 -> PwrSupplyOut/9  "Pwr_HV1toLV_max"
  PwrSupplyOut.Pwr_HV1toHV2_max/1 -> PwrSupplyOut/10  "Pwr_HV1toHV2_max"
  PwrSupplyOut.Eta_HV1toLV/1 -> PwrSupplyOut/11  "Eta_HV1toLV"
  PwrSupplyOut.Eta_HV1toHV2/1 -> PwrSupplyOut/12  "Eta_HV1toHV2"
  Trq_Supp2Bdy1/1 -> cmPowerTrainXWDOut/14  "Trq_Supp2Bdy1"
  Trq_Supp2Bdy1.rx/1 -> Trq_Supp2Bdy1/1  "rx"
  Trq_Supp2Bdy1.ry/1 -> Trq_Supp2Bdy1/2  "ry"
  Trq_Supp2Bdy1.rz/1 -> Trq_Supp2Bdy1/3  "rz"
  Trq_Supp2Bdy1B/1 -> cmPowerTrainXWDOut/15  "Trq_Supp2Bdy1B"
  Trq_Supp2Bdy1B.rx/1 -> Trq_Supp2Bdy1B/1  "rx"
  Trq_Supp2Bdy1B.ry/1 -> Trq_Supp2Bdy1B/2  "ry"
  Trq_Supp2Bdy1B.rz/1 -> Trq_Supp2Bdy1B/3  "rz"
  Trq_Supp2BdyEng/1 -> cmPowerTrainXWDOut/16  "Trq_Supp2BdyEng"
  Trq_Supp2BdyEng.rx/1 -> Trq_Supp2BdyEng/1  "rx"
  Trq_Supp2BdyEng.ry/1 -> Trq_Supp2BdyEng/2  "ry"
  DL_iDiff_mean/1 -> cmPowerTrainXWDOut/17  "DL_iDiff_mean"
  WheelOut/1 -> cmPowerTrainXWDOut/18  "WheelOut"
  WheelOut.FL/1 -> WheelOut/1  "FL"
  WheelOut.FL.Inert_in/1 -> WheelOut.FL/1  "Inert_in"
  WheelOut.FR/1 -> WheelOut/2  "FR"
  WheelOut.FR.Inert_in/1 -> WheelOut.FR/1  "Inert_in"
  WheelOut.RL/1 -> WheelOut/3  "RL"
  WheelOut.RL.Inert_in/1 -> WheelOut.RL/1  "Inert_in"
  WheelOut.RR/1 -> WheelOut/4  "RR"
  WheelOut.RR.Inert_in/1 -> WheelOut.RR/1  "Inert_in"
  PowerDelta/1 -> cmPowerTrainXWDOut/19  "PowerDelta"
  PowerDelta.PlanetGear/1 -> PowerDelta/1  "PlanetGear"
  PowerDelta.Diffs/1 -> PowerDelta/2  "Diffs"
  PowerDelta.Shafts/1 -> PowerDelta/3  "Shafts"
  PowerDelta.Spring_DL/1 -> PowerDelta/4  "Spring_DL"
  PowerDelta.Inert_DL/1 -> PowerDelta/5  "Inert_DL"
  PowerDelta.Inert/1 -> PowerDelta/6  "Inert"
  PowerDelta.PowerSupply/1 -> PowerDelta/7  "PowerSupply"
  WheelOut.FL.Trq_Drive/1 -> WheelOut.FL/2  "Trq_Drive"
  WheelOut.FL.Trq_Supp2WC/1 -> WheelOut.FL/3  "Trq_Supp2WC"
  WheelOut.FR.Trq_Drive/1 -> WheelOut.FR/2  "Trq_Drive"
  WheelOut.FR.Trq_Supp2WC/1 -> WheelOut.FR/3  "Trq_Supp2WC"
  WheelOut.RL.Trq_Drive/1 -> WheelOut.RL/2  "Trq_Drive"
  WheelOut.RL.Trq_Supp2WC/1 -> WheelOut.RL/3  "Trq_Supp2WC"
  WheelOut.RR.Trq_Drive/1 -> WheelOut.RR/2  "Trq_Drive"
  WheelOut.RR.Trq_Supp2WC/1 -> WheelOut.RR/3  "Trq_Supp2WC"

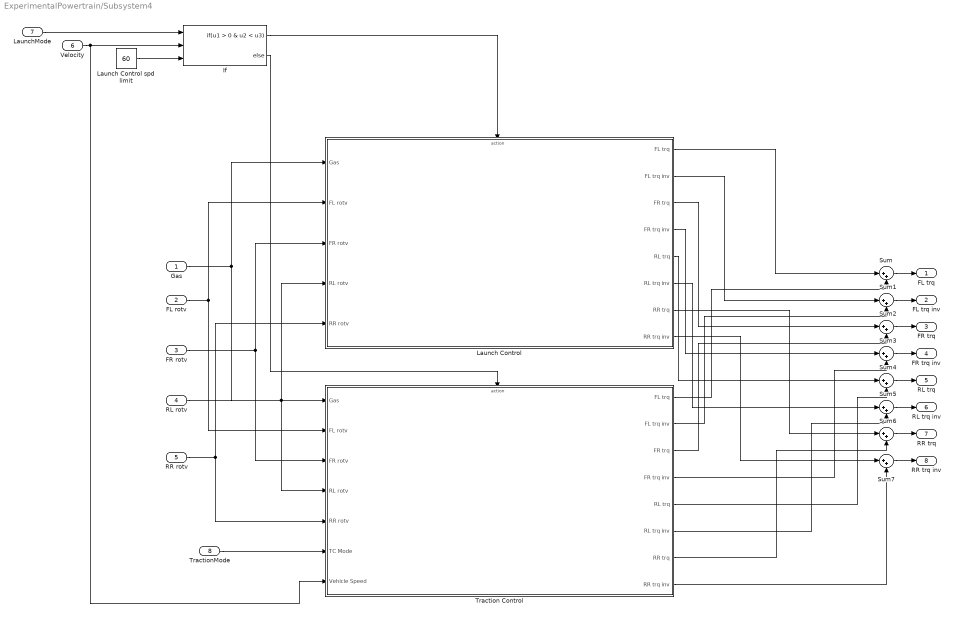
== system ExperimentalPowertrain/Subsystem4 ==
  Gas : Inport
  FL rotv : Inport  Port=2
  FR rotv : Inport  Port=3
  RL rotv : Inport  Port=4
  RR rotv : Inport  Port=5
  Velocity : Inport  Port=6
  LaunchMode : Inport  Port=7
  TractionMode : Inport  Port=8
  If : If  NumInputs=3  IfExpression=u1 > 0 & u2 < u3
  Launch Control : Subsystem  TreatAsAtomicUnit=on
  Launch Control spd limit : Constant  Value=60
  Sum{,1..7} (8 alike) : Sum  Inputs=|++
  Traction Control : Subsystem  TreatAsAtomicUnit=on
  FL trq : Outport
  FL trq inv : Outport  Port=2
  FR trq : Outport  Port=3
  FR trq inv : Outport  Port=4
  RL trq : Outport  Port=5
  RL trq inv : Outport  Port=6
  RR trq : Outport  Port=7
  RR trq inv : Outport  Port=8
  wires:
  Gas/1 -> Launch Control/1(Gas), Traction Control/1(Gas)
  FL rotv/1 -> Launch Control/2(FL rotv), Traction Control/2(FL rotv)
  FR rotv/1 -> Launch Control/3(FR rotv), Traction Control/3(FR rotv)
  RL rotv/1 -> Launch Control/4(RL rotv), Traction Control/4(RL rotv)
  RR rotv/1 -> Launch Control/5(RR rotv), Traction Control/5(RR rotv)
  LaunchMode/1 -> If/1
  Velocity/1 -> Traction Control/7(Vehicle Speed), If/2
  Launch Control spd limit/1 -> If/3
  If/1 -> Launch Control/Action
  If/2 -> Traction Control/Action
  Launch Control/1(FL trq) -> Sum/1
  Launch Control/2(FL trq inv) -> Sum1/1
  Launch Control/3(FR trq) -> Sum2/1
  Launch Control/4(FR trq inv) -> Sum3/1
  Launch Control/5(RL trq) -> Sum4/1
  Launch Control/6(RL trq inv) -> Sum5/1
  Launch Control/7(RR trq) -> Sum6/1
  Launch Control/8(RR trq inv) -> Sum7/1
  Sum/1 -> FL trq/1
  Sum1/1 -> FL trq inv/1
  Sum2/1 -> FR trq/1
  Sum3/1 -> FR trq inv/1
  Sum4/1 -> RL trq/1
  Sum5/1 -> RL trq inv/1
  Sum6/1 -> RR trq/1
  Sum7/1 -> RR trq inv/1
  Traction Control/1(FL trq) -> Sum/2
  Traction Control/2(FL trq inv) -> Sum1/2
  Traction Control/3(FR trq) -> Sum2/2
  Traction Control/4(FR trq inv) -> Sum3/2
  Traction Control/5(RL trq) -> Sum4/2
  Traction Control/6(RL trq inv) -> Sum5/2
  Traction Control/7(RR trq) -> Sum6/2
  Traction Control/8(RR trq inv) -> Sum7/2
  TractionMode/1 -> Traction Control/6(TC Mode)

== system ExperimentalPowertrain/Subsystem4/Launch Control ==
  Gas : Inport
  FL rotv : Inport  Port=2
  FR rotv : Inport  Port=3
  RL rotv : Inport  Port=4
  RR rotv : Inport  Port=5
  Action Port : ActionPort  ActionPortLabel=if(u1 > 0 & u2 < u3)
  LaunchControl : Subsystem
  FL trq : Outport
  FL trq inv : Outport  Port=2
  FR trq : Outport  Port=3
  FR trq inv : Outport  Port=4
  RL trq : Outport  Port=5
  RL trq inv : Outport  Port=6
  RR trq : Outport  Port=7
  RR trq inv : Outport  Port=8
  wires:
  Gas/1 -> LaunchControl/1(Gas)
  FL rotv/1 -> LaunchControl/2(FL rotv)
  FR rotv/1 -> LaunchControl/3(FR rotv)
  RL rotv/1 -> LaunchControl/4(RL rotv)
  RR rotv/1 -> LaunchControl/5(RR rotv)
  LaunchControl/1(FL trq) -> FL trq/1
  LaunchControl/2(FL trq inv) -> FL trq inv/1
  LaunchControl/3(FR trq) -> FR trq/1
  LaunchControl/4(FR trq inv) -> FR trq inv/1
  LaunchControl/5(RL trq) -> RL trq/1
  LaunchControl/6(RL trq inv) -> RL trq inv/1
  LaunchControl/7(RR trq) -> RR trq/1
  LaunchControl/8(RR trq inv) -> RR trq inv/1

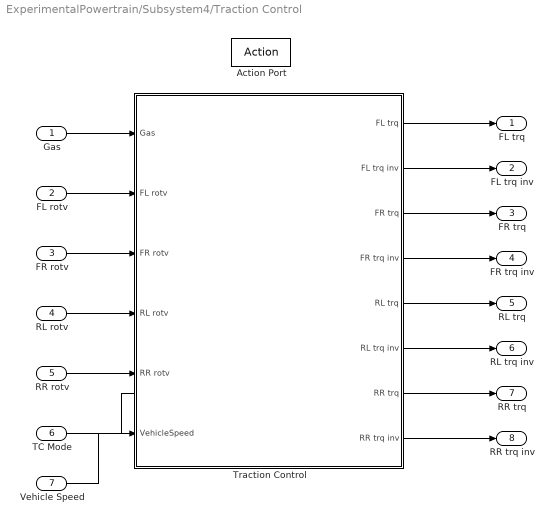
== system ExperimentalPowertrain/Subsystem4/Traction Control ==
  Gas : Inport
  FL rotv : Inport  Port=2
  FR rotv : Inport  Port=3
  RL rotv : Inport  Port=4
  RR rotv : Inport  Port=5
  TC Mode : Inport  Port=6
  Vehicle Speed : Inport  Port=7
  Action Port : ActionPort  ActionPortLabel=else
  Traction Control : Subsystem
  FL trq : Outport
  FL trq inv : Outport  Port=2
  FR trq : Outport  Port=3
  FR trq inv : Outport  Port=4
  RL trq : Outport  Port=5
  RL trq inv : Outport  Port=6
  RR trq : Outport  Port=7
  RR trq inv : Outport  Port=8
  wires:
  Gas/1 -> Traction Control/1(Gas)
  FL rotv/1 -> Traction Control/2(FL rotv)
  FR rotv/1 -> Traction Control/3(FR rotv)
  RL rotv/1 -> Traction Control/4(RL rotv)
  RR rotv/1 -> Traction Control/5(RR rotv)
  Traction Control/1(FL trq) -> FL trq/1
  Traction Control/2(FL trq inv) -> FL trq inv/1
  Traction Control/3(FR trq) -> FR trq/1
  Traction Control/4(FR trq inv) -> FR trq inv/1
  Traction Control/5(RL trq) -> RL trq/1
  Traction Control/6(RL trq inv) -> RL trq inv/1
  Traction Control/7(RR trq) -> RR trq/1
  Traction Control/8(RR trq inv) -> RR trq inv/1
  TC Mode/1 -> ?
  Vehicle Speed/1 -> Traction Control/6(VehicleSpeed)

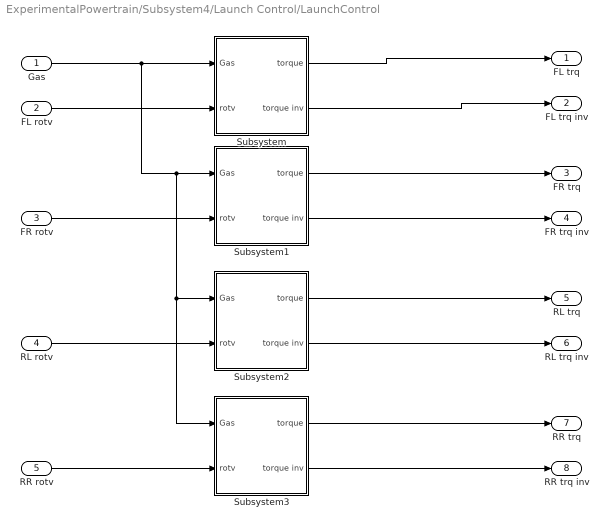
== system ExperimentalPowertrain/Subsystem4/Launch Control/LaunchControl ==
  Gas : Inport
  FL rotv : Inport  Port=2
  FR rotv : Inport  Port=3
  RL rotv : Inport  Port=4
  RR rotv : Inport  Port=5
  Subsystem : Subsystem
  Subsystem1 : Subsystem
  Subsystem2 : Subsystem
  Subsystem3 : Subsystem
  FL trq : Outport
  FL trq inv : Outport  Port=2
  FR trq : Outport  Port=3
  FR trq inv : Outport  Port=4
  RL trq : Outport  Port=5
  RL trq inv : Outport  Port=6
  RR trq : Outport  Port=7
  RR trq inv : Outport  Port=8
  wires:
  Subsystem1/1(torque) -> FR trq/1
  Gas/1 -> Subsystem1/1(Gas), Subsystem3/1(Gas), Subsystem2/1(Gas), Subsystem/1(Gas)
  Subsystem2/2(torque inv) -> RL trq inv/1
  RR rotv/1 -> Subsystem3/2(rotv)
  Subsystem1/2(torque inv) -> FR trq inv/1
  Subsystem3/1(torque) -> RR trq/1
  FR rotv/1 -> Subsystem1/2(rotv)
  Subsystem2/1(torque) -> RL trq/1
  RL rotv/1 -> Subsystem2/2(rotv)
  FL rotv/1 -> Subsystem/2(rotv)
  Subsystem/2(torque inv) -> FL trq inv/1
  Subsystem/1(torque) -> FL trq/1
  Subsystem3/2(torque inv) -> RR trq inv/1

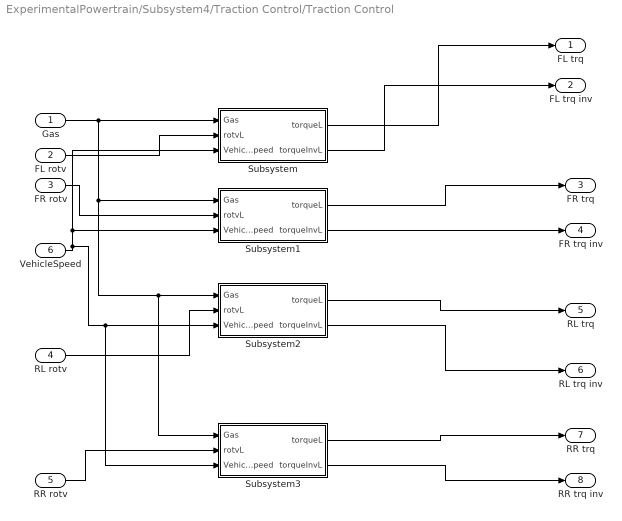
== system ExperimentalPowertrain/Subsystem4/Traction Control/Traction Control ==
  Gas : Inport
  FL rotv : Inport  Port=2
  FR rotv : Inport  Port=3
  RL rotv : Inport  Port=4
  RR rotv : Inport  Port=5
  VehicleSpeed : Inport  Port=6
  Subsystem : Subsystem
  Subsystem1 : Subsystem
  Subsystem2 : Subsystem
  Subsystem3 : Subsystem
  FL trq : Outport
  FL trq inv : Outport  Port=2
  FR trq : Outport  Port=3
  FR trq inv : Outport  Port=4
  RL trq : Outport  Port=5
  RL trq inv : Outport  Port=6
  RR trq : Outport  Port=7
  RR trq inv : Outport  Port=8
  wires:
  Gas/1 -> Subsystem1/1(Gas), Subsystem3/1(Gas), Subsystem2/1(Gas), Subsystem/1(Gas)
  FL rotv/1 -> Subsystem/2(rotvL)
  Subsystem/2(torqueInvL) -> FL trq inv/1
  Subsystem/1(torqueL) -> FL trq/1
  FR rotv/1 -> Subsystem1/2(rotvL)
  VehicleSpeed/1 -> Subsystem3/3(Vehicle Speed), Subsystem2/3(Vehicle Speed), Subsystem1/3(Vehicle Speed), Subsystem/3(Vehicle Speed)
  Subsystem1/1(torqueL) -> FR trq/1
  Subsystem1/2(torqueInvL) -> FR trq inv/1
  Subsystem2/1(torqueL) -> RL trq/1
  Subsystem2/2(torqueInvL) -> RL trq inv/1
  Subsystem3/1(torqueL) -> RR trq/1
  Subsystem3/2(torqueInvL) -> RR trq inv/1
  RL rotv/1 -> Subsystem2/2(rotvL)
  RR rotv/1 -> Subsystem3/2(rotvL)

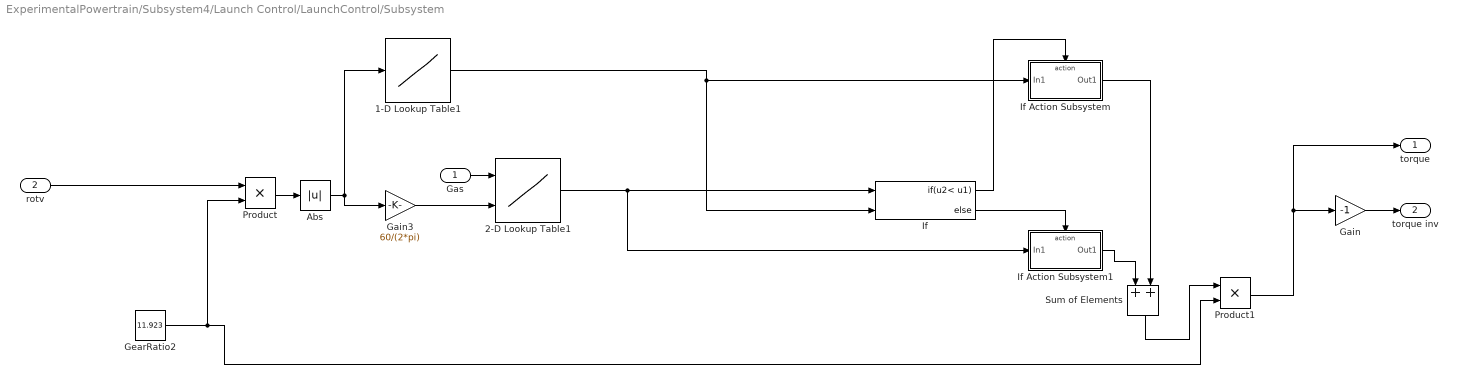
== system ExperimentalPowertrain/Subsystem4/Launch Control/LaunchControl/Subsystem ==
  Gas : Inport
  rotv : Inport  Port=2
  1-D Lookup Table1 : Lookup_n-D  NumberOfTableDimensions=1  BreakpointsForDimension1=[0 2000 4000 6000 8000 10000 12000 14000 15000 16000 17000 18000 20000 22000]  Table=[9 10 12 15 25 25 25 25 25 25 25 25 25 0]  InternalRulePriority=Speed  RndMeth=Simplest  InputSameDT=on
  2-D Lookup Table1 : Lookup_n-D  BreakpointsForDimension1=[0 0.2 0.4 0.6 0.8 1]  BreakpointsForDimension2=[0 2000 4000 6000 8000 10000 12000 14000 15000 16000 17000 18000 20000 22000]  Table=[0 0 0 0 0 0 0 0 0 0 0 0 0 0;4 4 4 4 4 4 4 4 4 4 4 4 3 0;8 8 8 8 8 8 8 8 8 8 8 8 6 0;13 13 13 13 13 13 13 13 13 12 12 11 9 0;17 17 17 17 17 17 17 17 17 16 16 15 12 0;21 21 21 21 21 21 21 21 21 20 20 19 15 0]  InternalRulePriority=Speed  RndMeth=Simplest  InputSameDT=on
  Abs : Abs
  Gain : Gain  Gain=-1
  Gain3 : Gain  Gain=60/(2*pi)
  GearRatio2 : Constant  Value=11.923
  If : If  NumInputs=2  IfExpression=u2< u1
  If Action Subsystem : Subsystem  TreatAsAtomicUnit=on
  If Action Subsystem1 : Subsystem  TreatAsAtomicUnit=on
  Product : Product
  Product1 : Product
  Sum of Elements : Sum  Inputs=2
  torque : Outport
  torque inv : Outport  Port=2
  wires:
  Gain/1 -> torque inv/1
  Abs/1 -> Gain3/1, 1-D Lookup Table1/1
  2-D Lookup Table1/1 -> If Action Subsystem1/1(In1), If/1
  1-D Lookup Table1/1 -> If/2, If Action Subsystem/1(In1)
  Product/1 -> Abs/1
  If/1 -> If Action Subsystem/Action
  If/2 -> If Action Subsystem1/Action
  If Action Subsystem/1(Out1) -> Sum of Elements/2
  If Action Subsystem1/1(Out1) -> Sum of Elements/1
  GearRatio2/1 -> Product/2, Product1/2
  Gain3/1 -> 2-D Lookup Table1/2
  Sum of Elements/1 -> Product1/1
  Product1/1 -> torque/1, Gain/1
  rotv/1 -> Product/1
  Gas/1 -> 2-D Lookup Table1/1

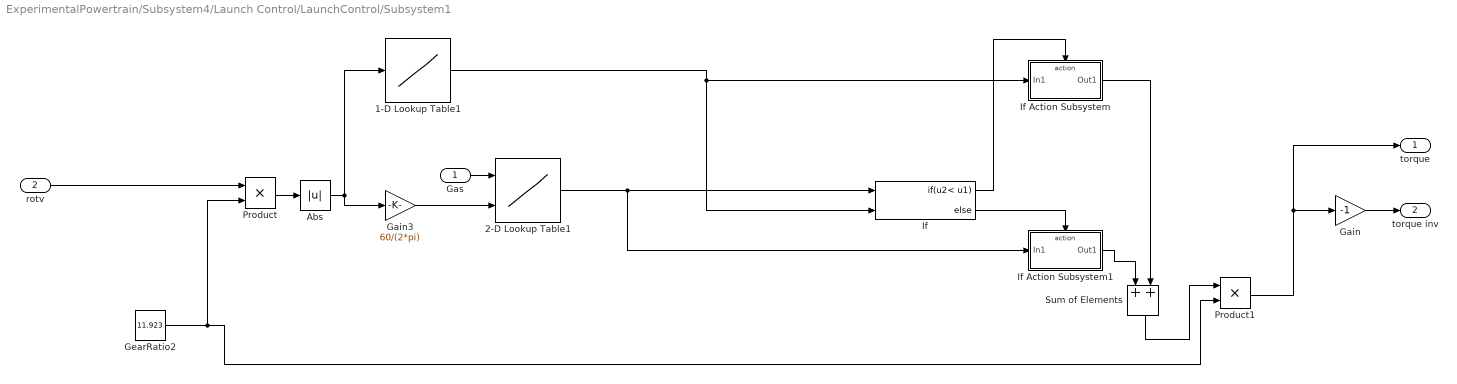
== system ExperimentalPowertrain/Subsystem4/Launch Control/LaunchControl/Subsystem1 ==
  Gas : Inport
  rotv : Inport  Port=2
  1-D Lookup Table1 : Lookup_n-D  NumberOfTableDimensions=1  BreakpointsForDimension1=[0 2000 4000 6000 8000 10000 12000 14000 15000 16000 17000 18000 20000 22000]  Table=[9 10 12 15 25 25 25 25 25 25 25 25 25 0]  InternalRulePriority=Speed  RndMeth=Simplest  InputSameDT=on
  2-D Lookup Table1 : Lookup_n-D  BreakpointsForDimension1=[0 0.2 0.4 0.6 0.8 1]  BreakpointsForDimension2=[0 2000 4000 6000 8000 10000 12000 14000 15000 16000 17000 18000 20000 22000]  Table=[0 0 0 0 0 0 0 0 0 0 0 0 0 0;4 4 4 4 4 4 4 4 4 4 4 4 3 0;8 8 8 8 8 8 8 8 8 8 8 8 6 0;13 13 13 13 13 13 13 13 13 12 12 11 9 0;17 17 17 17 17 17 17 17 17 16 16 15 12 0;21 21 21 21 21 21 21 21 21 20 20 19 15 0]  InternalRulePriority=Speed  RndMeth=Simplest  InputSameDT=on
  Abs : Abs
  Gain : Gain  Gain=-1
  Gain3 : Gain  Gain=60/(2*pi)
  GearRatio2 : Constant  Value=11.923
  If : If  NumInputs=2  IfExpression=u2< u1
  If Action Subsystem : Subsystem  TreatAsAtomicUnit=on
  If Action Subsystem1 : Subsystem  TreatAsAtomicUnit=on
  Product : Product
  Product1 : Product
  Sum of Elements : Sum  Inputs=2
  torque : Outport
  torque inv : Outport  Port=2
  wires:
  Gain/1 -> torque inv/1
  Abs/1 -> Gain3/1, 1-D Lookup Table1/1
  2-D Lookup Table1/1 -> If Action Subsystem1/1(In1), If/1
  1-D Lookup Table1/1 -> If/2, If Action Subsystem/1(In1)
  Product/1 -> Abs/1
  If/1 -> If Action Subsystem/Action
  If/2 -> If Action Subsystem1/Action
  If Action Subsystem/1(Out1) -> Sum of Elements/2
  If Action Subsystem1/1(Out1) -> Sum of Elements/1
  GearRatio2/1 -> Product/2, Product1/2
  Gain3/1 -> 2-D Lookup Table1/2
  Sum of Elements/1 -> Product1/1
  Product1/1 -> torque/1, Gain/1
  rotv/1 -> Product/1
  Gas/1 -> 2-D Lookup Table1/1

== system ExperimentalPowertrain/Subsystem4/Launch Control/LaunchControl/Subsystem2 ==
  Gas : Inport
  rotv : Inport  Port=2
  1-D Lookup Table1 : Lookup_n-D  NumberOfTableDimensions=1  BreakpointsForDimension1=[0 400 800 1200 1600 2000 3000 4000 6000 22000]  Table=[18 20 23 25 25 25 25 25 25 25]  InternalRulePriority=Speed  RndMeth=Simplest  InputSameDT=on
  2-D Lookup Table1 : Lookup_n-D  BreakpointsForDimension1=[0 0.2 0.4 0.6 0.8 1]  BreakpointsForDimension2=[0 2000 4000 6000 8000 10000 12000 14000 15000 16000 17000 18000 20000 22000]  Table=[0 0 0 0 0 0 0 0 0 0 0 0 0 0;4 4 4 4 4 4 4 4 4 4 4 4 3 0;8 8 8 8 8 8 8 8 8 8 8 8 6 0;13 13 13 13 13 13 13 13 13 12 12 11 9 0;17 17 17 17 17 17 17 17 17 16 16 15 12 0;21 21 21 21 21 21 21 21 21 20 20 19 15 0]  InternalRulePriority=Speed  RndMeth=Simplest  InputSameDT=on
  Abs : Abs
  Gain : Gain  Gain=-1
  Gain3 : Gain  Gain=60/(2*pi)
  GearRatio2 : Constant  Value=11.923
  If : If  NumInputs=2  IfExpression=u2< u1
  If Action Subsystem : Subsystem  TreatAsAtomicUnit=on
  If Action Subsystem1 : Subsystem  TreatAsAtomicUnit=on
  Product : Product
  Product1 : Product
  Sum of Elements : Sum  Inputs=2
  torque : Outport
  torque inv : Outport  Port=2
  wires:
  Gain/1 -> torque inv/1
  Abs/1 -> Gain3/1, 1-D Lookup Table1/1
  2-D Lookup Table1/1 -> If Action Subsystem1/1(In1), If/1
  1-D Lookup Table1/1 -> If/2, If Action Subsystem/1(In1)
  Product/1 -> Abs/1
  If/1 -> If Action Subsystem/Action
  If/2 -> If Action Subsystem1/Action
  If Action Subsystem/1(Out1) -> Sum of Elements/2
  If Action Subsystem1/1(Out1) -> Sum of Elements/1
  GearRatio2/1 -> Product/2, Product1/2
  Gain3/1 -> 2-D Lookup Table1/2
  Sum of Elements/1 -> Product1/1
  Product1/1 -> torque/1, Gain/1
  rotv/1 -> Product/1
  Gas/1 -> 2-D Lookup Table1/1

== system ExperimentalPowertrain/Subsystem4/Launch Control/LaunchControl/Subsystem3 ==
  Gas : Inport
  rotv : Inport  Port=2
  1-D Lookup Table1 : Lookup_n-D  NumberOfTableDimensions=1  BreakpointsForDimension1=[0 400 800 1200 1600 2000 3000 4000 6000 22000]  Table=[18 20 23 25 25 25 25 25 25 25]  InternalRulePriority=Speed  RndMeth=Simplest  InputSameDT=on
  2-D Lookup Table1 : Lookup_n-D  BreakpointsForDimension1=[0 0.2 0.4 0.6 0.8 1]  BreakpointsForDimension2=[0 2000 4000 6000 8000 10000 12000 14000 15000 16000 17000 18000 20000 22000]  Table=[0 0 0 0 0 0 0 0 0 0 0 0 0 0;4 4 4 4 4 4 4 4 4 4 4 4 3 0;8 8 8 8 8 8 8 8 8 8 8 8 6 0;13 13 13 13 13 13 13 13 13 12 12 11 9 0;17 17 17 17 17 17 17 17 17 16 16 15 12 0;21 21 21 21 21 21 21 21 21 20 20 19 15 0]  InternalRulePriority=Speed  RndMeth=Simplest  InputSameDT=on
  Abs : Abs
  Gain : Gain  Gain=-1
  Gain3 : Gain  Gain=60/(2*pi)
  GearRatio2 : Constant  Value=11.923
  If : If  NumInputs=2  IfExpression=u2< u1
  If Action Subsystem : Subsystem  TreatAsAtomicUnit=on
  If Action Subsystem1 : Subsystem  TreatAsAtomicUnit=on
  Product : Product
  Product1 : Product
  Sum of Elements : Sum  Inputs=2
  torque : Outport
  torque inv : Outport  Port=2
  wires:
  Gain/1 -> torque inv/1
  Abs/1 -> Gain3/1, 1-D Lookup Table1/1
  2-D Lookup Table1/1 -> If Action Subsystem1/1(In1), If/1
  1-D Lookup Table1/1 -> If/2, If Action Subsystem/1(In1)
  Product/1 -> Abs/1
  If/1 -> If Action Subsystem/Action
  If/2 -> If Action Subsystem1/Action
  If Action Subsystem/1(Out1) -> Sum of Elements/2
  If Action Subsystem1/1(Out1) -> Sum of Elements/1
  GearRatio2/1 -> Product/2, Product1/2
  Gain3/1 -> 2-D Lookup Table1/2
  Sum of Elements/1 -> Product1/1
  Product1/1 -> torque/1, Gain/1
  rotv/1 -> Product/1
  Gas/1 -> 2-D Lookup Table1/1

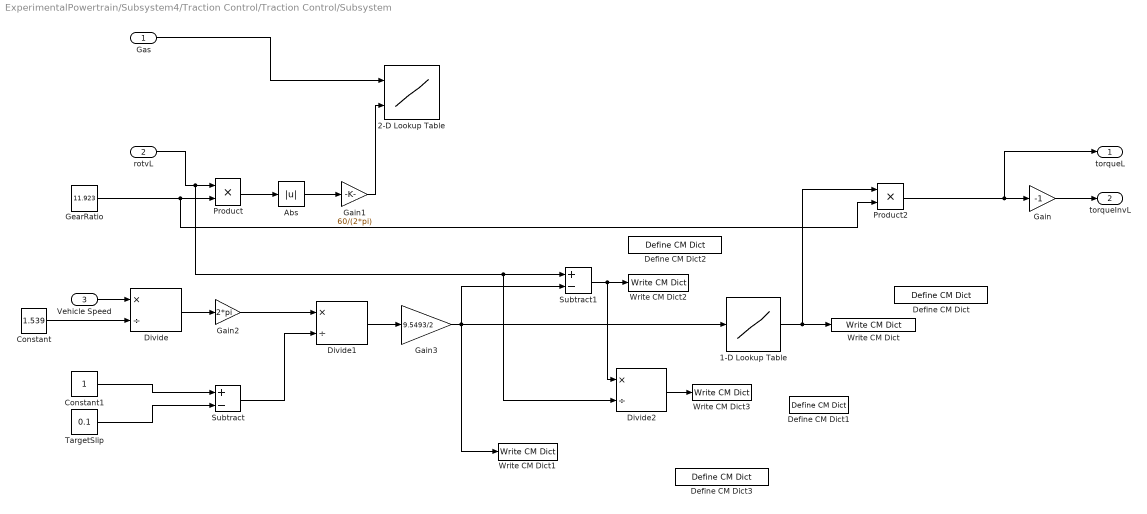
== system ExperimentalPowertrain/Subsystem4/Traction Control/Traction Control/Subsystem ==
  Gas : Inport
  rotvL : Inport  Port=2
  Vehicle Speed : Inport  Port=3
  1-D Lookup Table : Lookup_n-D  NumberOfTableDimensions=1  BreakpointsForDimension1=[0 2000 4000 6000 8000 10000 12000 14000 15000 16000 17000 18000 20000 22000]  Table=[21 21 21 21 21 21 21 21 21 20 20 19 15 0]  InternalRulePriority=Speed  RndMeth=Simplest  InputSameDT=on
  2-D Lookup Table : Lookup_n-D  BreakpointsForDimension1=[0 0.2 0.4 0.6 0.8 1]  BreakpointsForDimension2=[0 2000 4000 6000 8000 10000 12000 14000 15000 16000 17000 18000 20000 22000]  Table=[0 0 0 0 0 0 0 0 0 0 0 0 0 0;4 4 4 4 4 4 4 4 4 4 4 4 3 0;8 8 8 8 8 8 8 8 8 8 8 8 6 0;13 13 13 13 13 13 13 13 13 12 12 11 9 0;17 17 17 17 17 17 17 17 17 16 16 15 12 0;21 21 21 21 21 21 21 21 21 20 20 19 15 0]  InternalRulePriority=Speed  RndMeth=Simplest  InputSameDT=on
  Abs : Abs
  Constant : Constant  Value=1.539
  Constant1 : Constant
  Define CM Dict : CarMaker4SL/Define CM Dict  xname=Caleb.TorqueTarget  xmono=off  xtype=Double4  xdvaplace=None  xnstates=0  xfirststate=0  xinitial=0
  Define CM Dict1 : CarMaker4SL/Define CM Dict  xname=Caleb.FrontTarget  xmono=off  xtype=Double4  xdvaplace=None  xnstates=0  xfirststate=0  xinitial=0
  Define CM Dict2 : CarMaker4SL/Define CM Dict  xname=Caleb.RotDiff  xmono=off  xtype=Double4  xdvaplace=None  xnstates=0  xfirststate=0  xinitial=0
  Define CM Dict3 : CarMaker4SL/Define CM Dict  xname=Caleb.PerDiff  xmono=off  xtype=Double4  xdvaplace=None  xnstates=0  xfirststate=0  xinitial=0
  Divide : Product  Inputs=*/
  Divide1 : Product  Inputs=*/
  Divide2 : Product  Inputs=*/
  Gain : Gain  Gain=-1
  Gain1 : Gain  Gain=60/(2*pi)
  Gain2 : Gain  Gain=2*pi
  Gain3 : Gain  Gain=9.5493/2
  GearRatio : Constant  Value=11.923
  Product : Product
  Product2 : Product
  Subtract : Sum  Inputs=+-
  Subtract1 : Sum  Inputs=+-
  TargetSlip : Constant  Value=0.1
  Write CM Dict : CarMaker4SL/Write CM Dict  xname=Caleb.TorqueTarget  xsync=off
  Write CM Dict1 : CarMaker4SL/Write CM Dict  xname=Caleb.FrontTarget  xsync=off
  Write CM Dict2 : CarMaker4SL/Write CM Dict  xname=Caleb.RotDiff  xsync=off
  Write CM Dict3 : CarMaker4SL/Write CM Dict  xname=Caleb.PerDiff  xsync=off
  torqueL : Outport
  torqueInvL : Outport  Port=2
  wires:
  Gain/1 -> torqueInvL/1
  Product/1 -> Abs/1
  Gas/1 -> 2-D Lookup Table/1
  GearRatio/1 -> Product2/2, Product/2
  rotvL/1 -> Divide2/2, Subtract1/1, Product/1
  Product2/1 -> Gain/1, torqueL/1
  Abs/1 -> Gain1/1
  Gain1/1 -> 2-D Lookup Table/2
  TargetSlip/1 -> Subtract/2
  Vehicle Speed/1 -> Divide/1
  Constant/1 -> Divide/2
  Divide/1 -> Gain2/1
  Gain2/1 -> Divide1/1
  Constant1/1 -> Subtract/1
  Subtract/1 -> Divide1/2
  Divide1/1 -> Gain3/1
  Gain3/1 -> Write CM Dict1/1, Subtract1/2, 1-D Lookup Table/1
  1-D Lookup Table/1 -> Product2/1, Write CM Dict/1
  Subtract1/1 -> Divide2/1, Write CM Dict2/1
  Divide2/1 -> Write CM Dict3/1

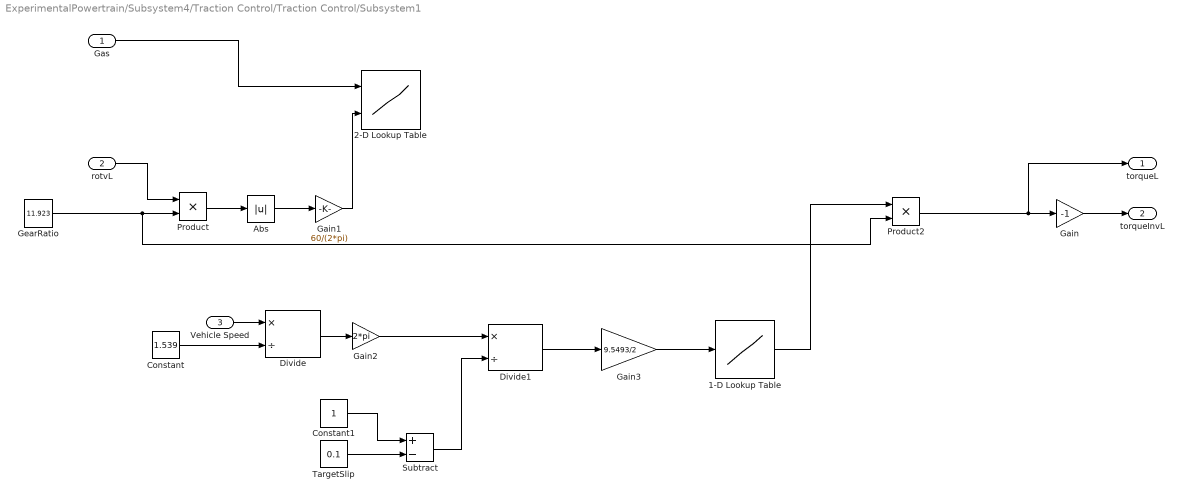
== system ExperimentalPowertrain/Subsystem4/Traction Control/Traction Control/Subsystem1 ==
  Gas : Inport
  rotvL : Inport  Port=2
  Vehicle Speed : Inport  Port=3
  1-D Lookup Table : Lookup_n-D  NumberOfTableDimensions=1  BreakpointsForDimension1=[0 2000 4000 6000 8000 10000 12000 14000 15000 16000 17000 18000 20000 22000]  Table=[21 21 21 21 21 21 21 21 21 20 20 19 15 0]  InternalRulePriority=Speed  RndMeth=Simplest  InputSameDT=on
  2-D Lookup Table : Lookup_n-D  BreakpointsForDimension1=[0 0.2 0.4 0.6 0.8 1]  BreakpointsForDimension2=[0 2000 4000 6000 8000 10000 12000 14000 15000 16000 17000 18000 20000 22000]  Table=[0 0 0 0 0 0 0 0 0 0 0 0 0 0;4 4 4 4 4 4 4 4 4 4 4 4 3 0;8 8 8 8 8 8 8 8 8 8 8 8 6 0;13 13 13 13 13 13 13 13 13 12 12 11 9 0;17 17 17 17 17 17 17 17 17 16 16 15 12 0;21 21 21 21 21 21 21 21 21 20 20 19 15 0]  InternalRulePriority=Speed  RndMeth=Simplest  InputSameDT=on
  Abs : Abs
  Constant : Constant  Value=1.539
  Constant1 : Constant
  Divide : Product  Inputs=*/
  Divide1 : Product  Inputs=*/
  Gain : Gain  Gain=-1
  Gain1 : Gain  Gain=60/(2*pi)
  Gain2 : Gain  Gain=2*pi
  Gain3 : Gain  Gain=9.5493/2
  GearRatio : Constant  Value=11.923
  Product : Product
  Product2 : Product
  Subtract : Sum  Inputs=+-
  TargetSlip : Constant  Value=0.1
  torqueL : Outport
  torqueInvL : Outport  Port=2
  wires:
  Gain/1 -> torqueInvL/1
  Product/1 -> Abs/1
  Gas/1 -> 2-D Lookup Table/1
  GearRatio/1 -> Product2/2, Product/2
  rotvL/1 -> Product/1
  Product2/1 -> Gain/1, torqueL/1
  Abs/1 -> Gain1/1
  Gain1/1 -> 2-D Lookup Table/2
  TargetSlip/1 -> Subtract/2
  Vehicle Speed/1 -> Divide/1
  Constant/1 -> Divide/2
  Divide/1 -> Gain2/1
  Gain2/1 -> Divide1/1
  Constant1/1 -> Subtract/1
  Subtract/1 -> Divide1/2
  Divide1/1 -> Gain3/1
  Gain3/1 -> 1-D Lookup Table/1
  1-D Lookup Table/1 -> Product2/1
